simulink model "nestedloop_simulation_jobmei"  (R2017a)
settings: Solver=FixedStepAuto  StartTime=0.0  StopTime=5  FixedStep=SampleTime  RelTol=1e-3
values from neighbouring files (symbols this model uses):
  C1 = H1_gain*H1_notch*H1_pd*H1_LP    [model_estimation.m]    (also in nestedloop_script.m)
  C21 = H21_gain*H21_notch*H21_LP1*H21_LP2*H21_I    [model_estimation.m]    (also in nestedloop_script.m)
  CFF = tf([1],[1])    [simulation_singlecontroller.m]
  H1 = H1_plant*sysdelay    [model_estimation.m]    (also in model_fitting.m; nestedloop_script.m; simulation_singlecontroller.m)
  H21 = H21_plant*sysdelay    [model_estimation.m]    (also in model_fitting.m; nestedloop_script.m; simulation_singlecontroller.m)
  SampleTime = 1/SampleRate    (= 0.00048828125)    [encoderTfEst.m]    (also in model_estimation.m; model_fitting.m; nestedloop_script.m; simulation_singlecontroller.m)
settings Model: Creator=marce  LastModifiedBy=marce

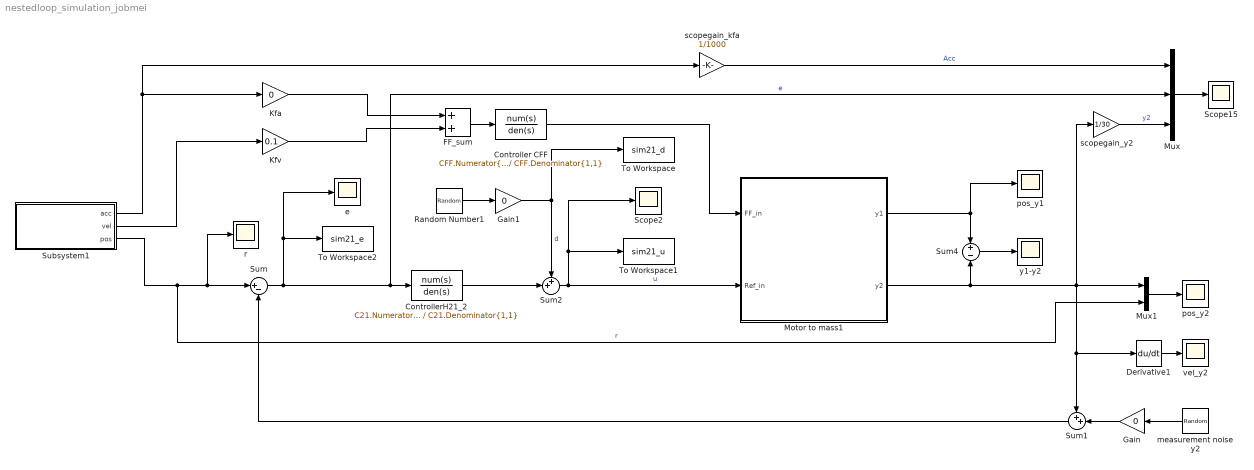
== system nestedloop_simulation_jobmei ==
  Controller CFF : TransferFcn  Numerator=CFF.Numerator{1,1}  Denominator=CFF.Denominator{1,1}
  ControllerH21_2 : TransferFcn  Numerator=C21.Numerator{1,1}  Denominator=C21.Denominator{1,1}
  Derivative1 : Derivative
  "FF_sum " : Sum
  Gain : Gain  Gain=0
  Gain1 : Gain  Gain=0
  Kfa : Gain  Gain=0
  Kfv : Gain  Gain=0.1
  Motor to mass1 : Subsystem
  Mux : Mux  Inputs=3
  Mux1 : Mux  Inputs=2
  Random Number1 : RandomNumber  SampleTime=SampleTime
  Scope15 : Scope
  Scope2 : Scope
  Subsystem1 : Subsystem  mask(Ref3){}
      settings: OpenFcn=r3g_main
      mask Display: disp('Ref3');
  Sum : Sum  Inputs=|+-
  Sum1 : Sum  Inputs=++|
  Sum2 : Sum  Inputs=++|
  Sum4 : Sum  Inputs=+|-
  To Workspace : ToWorkspace  VariableName=sim21_d  SaveFormat=Timeseries  SampleTime=-1
  To Workspace1 : ToWorkspace  VariableName=sim21_u  SaveFormat=Timeseries  SampleTime=-1
  To Workspace2 : ToWorkspace  VariableName=sim21_e  SaveFormat=Timeseries  SampleTime=-1
  e : Scope
  measurement noise y2 : RandomNumber  SampleTime=SampleTime
  pos_y1 : Scope
  pos_y2 : Scope
  r : Scope
  scopegain_kfa : Gain  Gain=1/1000
  scopegain_y2 : Gain  Gain=1/30
  vel_y2 : Scope
  y1-y2 : Scope
  wires:
  measurement noise y2/1 -> Gain/1
  Gain/1 -> Sum1/2
  Random Number1/1 -> Gain1/1
  Sum2/1 -> Motor to mass1/2("Ref_in "), Scope2/1, To Workspace1/1  "u"
  Gain1/1 -> Sum2/1, To Workspace/1  "d"
  Subsystem1/3(pos) -> Mux1/2, Sum/1, r/1  "r"
  Sum/1 -> Mux/2, ControllerH21_2/1, e/1, To Workspace2/1  "e"
  ControllerH21_2/1 -> Sum2/2
  Derivative1/1 -> vel_y2/1
  Sum1/1 -> Sum/2
  Motor to mass1/1(y1) -> Sum4/1, pos_y1/1
  Sum4/1 -> y1-y2/1
  Kfa/1 -> "FF_sum "/1
  Subsystem1/1(acc) -> Kfa/1, scopegain_kfa/1
  "FF_sum "/1 -> Controller CFF/1
  Kfv/1 -> "FF_sum "/2
  Subsystem1/2(vel) -> Kfv/1
  Mux/1 -> Scope15/1
  scopegain_kfa/1 -> Mux/1  "Acc"
  Motor to mass1/2(y2) -> scopegain_y2/1, Mux1/1, Sum1/1, Derivative1/1, Sum4/2
  scopegain_y2/1 -> Mux/3  "y2"
  Controller CFF/1 -> Motor to mass1/1(FF_in)
  Mux1/1 -> pos_y2/1

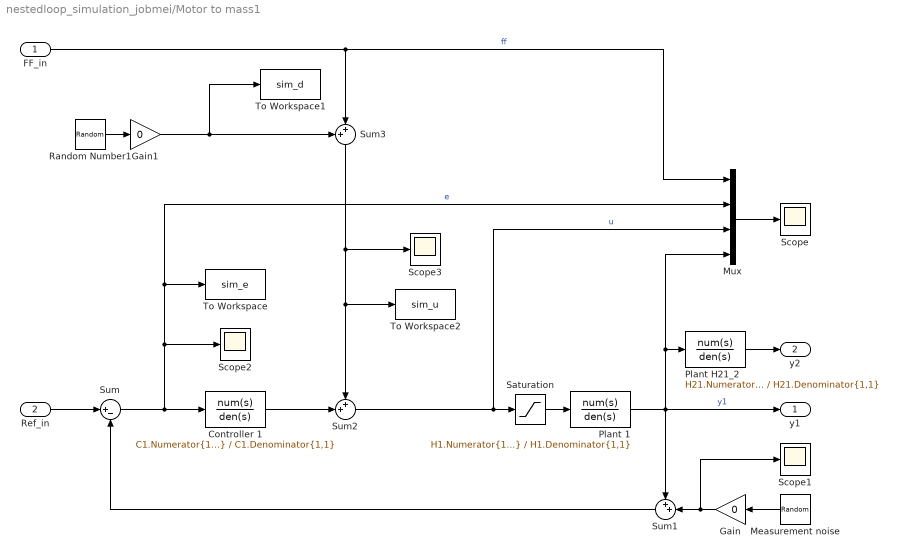
== system nestedloop_simulation_jobmei/Motor to mass1 ==
  FF_in : Inport
  "Ref_in " : Inport  Port=2
  Controller 1 : TransferFcn  Numerator=C1.Numerator{1,1}  Denominator=C1.Denominator{1,1}
  Gain : Gain  Gain=0
  Gain1 : Gain  Gain=0
  Measurement noise : RandomNumber  Variance=2  SampleTime=SampleTime
  Mux : Mux
  Plant 1 : TransferFcn  Numerator=H1.Numerator{1,1}  Denominator=H1.Denominator{1,1}
  Plant H21_2 : TransferFcn  Numerator=H21.Numerator{1,1}  Denominator=H21.Denominator{1,1}
  Random Number1 : RandomNumber  SampleTime=SampleTime
  Saturation : Saturate  UpperLimit=2.5  LowerLimit=-2.5
  Scope{,1..3} (4 alike) : Scope
  Sum : Sum  Inputs=|+-
  Sum1 : Sum  Inputs=++|
  Sum2 : Sum  Inputs=++|
  Sum3 : Sum  Inputs=++|
  To Workspace : ToWorkspace  VariableName=sim_e  SaveFormat=Timeseries  SampleTime=-1
  To Workspace1 : ToWorkspace  VariableName=sim_d  SaveFormat=Timeseries  SampleTime=-1
  To Workspace2 : ToWorkspace  VariableName=sim_u  SaveFormat=Timeseries  SampleTime=-1
  y1 : Outport
  y2 : Outport  Port=2
  wires:
  Gain1/1 -> To Workspace1/1, Sum3/1
  Measurement noise/1 -> Gain/1
  Gain/1 -> Sum1/2, Scope1/1
  Controller 1/1 -> Sum2/2
  Random Number1/1 -> Gain1/1
  "Ref_in "/1 -> Sum/1
  Sum1/1 -> Sum/2
  Sum/1 -> Scope2/1, Mux/2, To Workspace/1, Controller 1/1  "e"
  Saturation/1 -> Plant 1/1
  Plant 1/1 -> y1/1, Plant H21_2/1, Mux/4, Sum1/1  "y1"
  Plant H21_2/1 -> y2/1
  Sum2/1 -> Mux/3, Saturation/1  "u"
  Sum3/1 -> To Workspace2/1, Sum2/1, Scope3/1
  Mux/1 -> Scope/1
  FF_in/1 -> Mux/1, Sum3/2  "ff"

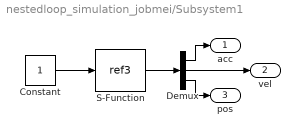
== system nestedloop_simulation_jobmei/Subsystem1 ==
  Constant : Constant
  Demux : Demux  Outputs=3
  S-Function : S-Function  FunctionName=ref3  Parameters=ref_part  SFunctionDeploymentMode=off  EnableBusSupport=off
      settings: OpenFcn=global ref_part; r3g_main
  acc : Outport
  vel : Outport  Port=2
  pos : Outport  Port=3
  wires:
  Constant/1 -> S-Function/1
  S-Function/1 -> Demux/1
  Demux/1 -> acc/1
  Demux/2 -> vel/1
  Demux/3 -> pos/1
